simulink model "LAB_02_26_SEPT_SIM_PENDOLO"  (R2022b)
settings: Solver=FixedStepAuto  StartTime=t0  StopTime=tf  FixedStep=0.1  MaxStep=0.2  RelTol=1e-3
values from neighbouring files (symbols this model uses):
  g = 9.81    [LAB_02_26_SEPT_MAT_PENDULUM.m]
  l = strcat([h,'',i])    [LAB_01_19_SEPT.m]    (also in LAB_02_26_SEPT_MAT_PENDULUM.m = 5)
  theta0 = 0    [LAB_02_26_SEPT_MAT_PENDULUM.m]    (also in LAB_05_24_OCT_MAT_KIN_COSDIR.m = 0.785398163397)
  theta_dot0 = pi/4    (= 0.785398163397)    [LAB_02_26_SEPT_MAT_PENDULUM.m]
settings Model: Creator=maria  LastModifiedBy=maria

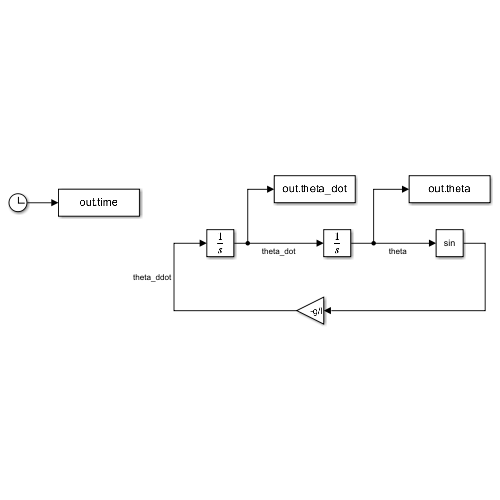
[thumbnail: Simulink's stored preview of the top-level diagram]
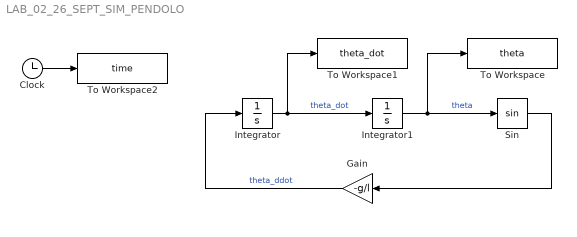
== system LAB_02_26_SEPT_SIM_PENDOLO ==
  Clock : Clock
  Gain : Gain  Gain=-g/l
  Integrator : Integrator  InitialCondition=theta_dot0
  Integrator1 : Integrator  InitialCondition=theta0
  Sin : Trigonometry
  To Workspace : ToWorkspace  VariableName=theta  SampleTime=-1
  To Workspace1 : ToWorkspace  VariableName=theta_dot  SampleTime=-1
  To Workspace2 : ToWorkspace  VariableName=time  SampleTime=-1
  wires:
  Integrator/1 -> To Workspace1/1, Integrator1/1  "theta_dot"
  Gain/1 -> Integrator/1  "theta_ddot"
  Integrator1/1 -> To Workspace/1, Sin/1  "theta"
  Sin/1 -> Gain/1
  Clock/1 -> To Workspace2/1
